simulink model "LCTC_vTD8_Test_TC0_ref6_2007a"  (Simulink 7.0)
settings: Solver=ode4  StartTime=0.0  StopTime=110  FixedStep=0.01  RelTol=1e-3
InitFcn:
  | PedalInterp_para
values from neighbouring files (symbols this model uses):
  ped_min = 5    [PedalInterp_para.m]
  T_max_Brake = 4000    [PedalInterp_para.m]
  TI = 0    [PAS_callback.m]
undefined symbols (not defined in the file or in its folder): fzgbib, m_ab_100pro, m_ab_70pro, PedalInterpretation, v_bereich
libraries: simulink x320
(part 1 of 23)
settings Model: Creator=Justyna  LastModifiedBy=Administrator  ExtModeAutoUpdateStatusClock=off
settings DataIOCC: SaveFormat=StructureWithTime  OutputSaveName=ZZZ
settings DebuggingCC: SaveWithParameterizedLinksMsg=none  SignalResolutionControl=TryResolveAllWithWarning  MultiTaskDSMMsg=warning  MultiTaskCondExecSysMsg=none  StrictBusMsg=None
settings HardwareCC: TargetHWDeviceType=32-bit Generic
settings RTWCC: IncludeERTFirstTime=on
settings GRTTargetCC: TargetFcnLib=ansi_tfl_tmw.mat

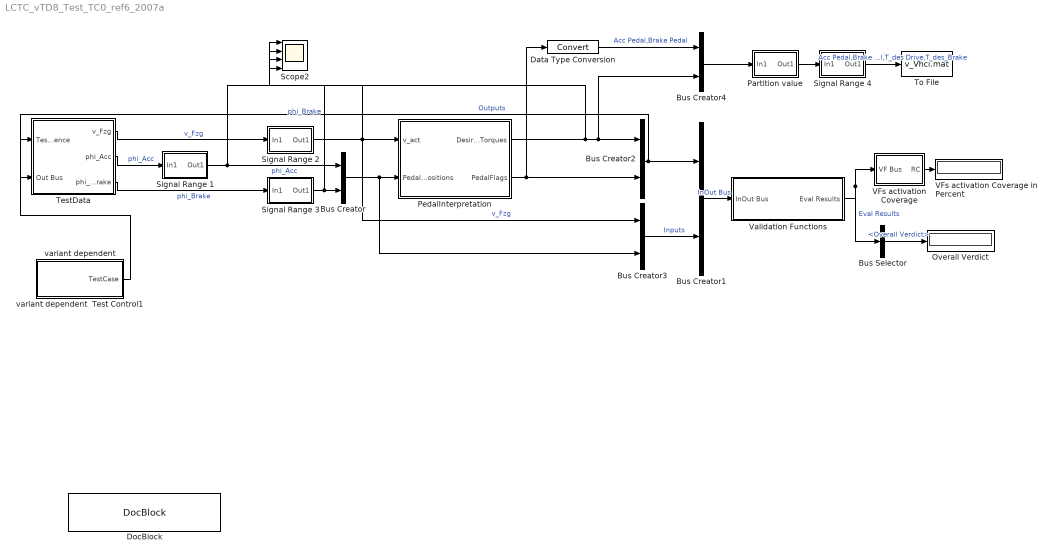
== system LCTC_vTD8_Test_TC0_ref6_2007a ==
  Bus Creator{,1..4} (5 alike) : BusCreator  Inputs=2
  Bus Selector : BusSelector  OutputSignals=Overall Verdict
  Data Type Conversion : DataTypeConversion  OutDataType=sfix(16)  OutScaling=2^0
  DocBlock : simulink/Model-Wide Utilities/DocBlock  SystemSampleTime=-1  DocumentType=Text
      content=|
      | jza - 21.08.07
      | The test model is created manually.
      |
      | Transformation rules for test data variants generation that should be implemented to obtain such a test model automatically are:
      | - for each set of generated variants a Stateflow should be added from the MIL Library: Test Data: Feature generation: Generate feature variants: TestDataVariantsSequence
      | - the number of states (with changed parameters)within TestDataVariantsSequence depends on the number of variants, so the states should be added if missing
      | - after(..) statement within TestDataVariantsSequence should be there as well, however we assume that the time value will be done manually (the same like in the case of independent test control)
      | - please note, that Generate limited increase and Generate limited decrease have been changed, however the same names and the same parameters are used. Probably, there will be no/less adjustment in the current version of transformation.
      | - SR block must contain such kind of brackets [x,y] instad of (x,y)
      |
      | jza - 14.09.07
      | corrections:
      | - switch in variants has a wrong condition - it should be u~=0,
      | - the number in a constant in variants does not work well - it worked for 2, for 3, but not for 4.
      | - time should be a parameter for: td variants, precondition duration, ingredient of test case duration in test control, ingredient of execution time
      | - constant in td have still boolean data type, although it should be "inherited from constant"
  "Overall Verdict   " : Display
  Partition value : Subsystem  mask{sr=[[],[],[0],[0]]}
      mask prompts: sr "signal range"
      mask help: Set the signal range for the input signals. The formal of range is (lower, upper). Lower stands for setting the minimum value of the input signal. Upper stands for setting the maximum value of the input signal. For example (-10,10)
      mask Display: fprintf('SR')
  PedalInterpretation : Subsystem  AncestorBlock=fzgbib/PedalInterpretation
      mask Display: fprintf('SUT')
  Scope2 : Scope  NumInputPorts=4
      settings: TimeRange=72  YMin=0~0~0~0.646597  YMax=70~0.275~27.5~0.908377  SaveName=ScopeData12  MaxDataPoints=11115000
  Signal Range 1 : Subsystem  mask{sr='[0,100]{}'}
      mask prompts: sr "signal range"
      mask help: Set the signal range for the input signals. The formal of range is (lower, upper). Lower stands for setting the minimum value of the input signal. Upper stands for setting the maximum value of the input signal. For example (-10,10)
      mask Display: fprintf('SR')
  Signal Range 2 : Subsystem  mask{sr='[-10,70]{0}'}
      mask prompts: sr "signal range"
      mask help: Set the signal range for the input signals. The formal of range is (lower, upper). Lower stands for setting the minimum value of the input signal. Upper stands for setting the maximum value of the input signal. For example (-10,10)
      mask Display: fprintf('SR')
  Signal Range 3 : Subsystem  mask{sr='[0,100]{}'}
      mask prompts: sr "signal range"
      mask help: Set the signal range for the input signals. The formal of range is (lower, upper). Lower stands for setting the minimum value of the input signal. Upper stands for setting the maximum value of the input signal. For example (-10,10)
      mask Display: fprintf('SR')
  Signal Range 4 : Subsystem  mask{sr=[[0,1],[0,1],[-8000,2300],[0,4000]]}
      mask prompts: sr "signal range"
      mask help: Set the signal range for the input signals. The formal of range is (lower, upper). Lower stands for setting the minimum value of the input signal. Upper stands for setting the maximum value of the input signal. For example (-10,10)
      mask Display: fprintf('SR')
  TestData : Subsystem
  To File : ToFile  Filename=v_Vhcl.mat  MatrixName=v_Vhcl
  VFs activation Coverage : Subsystem  mask{req=11, So=on}
      mask prompts: req "Number of Evaluated Scenarios within Requirements"; So "Adjust to the present Eva Results"
      mask StyleString: popup(1|2|3|4|5|6|7|8|9|10|11|12|13|14|15|16|17|18|19|20),checkbox
      mask CallbackString: |Requirements_Coverage_callback(gcb,-1)
  VFs activation Coverage in Percent : Display
  Validation Functions : Subsystem
  variant dependent : Subsystem  Orientation=left
  variant dependent  Test Control1 : Subsystem
  wires:
  PedalInterpretation/1(DesiredTorques) -> Scope2/3, Bus Creator2/1, Bus Creator4/2
  Bus Creator/1 -> PedalInterpretation/2(PedalPositions), Bus Creator3/2
  PedalInterpretation/2(PedalFlags) -> Bus Creator2/2, Data Type Conversion/1
  Validation Functions/1(Eval Results) -> VFs activation Coverage/1(VF Bus), Bus Selector/1  "Eval Results"
  Bus Creator1/1 -> Validation Functions/1(InOut Bus)  "InOut Bus"
  Bus Creator2/1 -> Bus Creator1/1, TestData/2(Out Bus)  "Outputs"
  Bus Creator3/1 -> Bus Creator1/2  "Inputs"
  VFs activation Coverage/1(RC) -> VFs activation Coverage in Percent/1
  Bus Selector/1 -> "Overall Verdict   "/1  "<Overall Verdict>"
  Signal Range 1/1(Out1) -> Bus Creator/1, Scope2/2  "phi_Acc"
  Signal Range 2/1(Out1) -> PedalInterpretation/1("v_act "), Bus Creator3/1, Scope2/1  "v_Fzg"
  Signal Range 3/1(Out1) -> Bus Creator/2, Scope2/4  "phi_Brake"
  Bus Creator4/1 -> Partition value/1(In1)
  Data Type Conversion/1 -> Bus Creator4/1  "Acc Pedal,Brake Pedal"
  Signal Range 4/1(Out1) -> To File/1  "Acc Pedal,Brake Pedal,T_des Drive,T_des_Brake"
  Partition value/1(Out1) -> Signal Range 4/1(In1)
  TestData/1(v_Fzg) -> Signal Range 2/1(In1)  "v_Fzg"
  TestData/2(phi_Acc) -> Signal Range 1/1(In1)  "phi_Acc"
  TestData/3(phi_Brake) -> Signal Range 3/1(In1)  "phi_Brake"
  variant dependent  Test Control1/1(TestCase) -> TestData/1(Test Ctrl Influence)

== system LCTC_vTD8_Test_TC0_ref6_2007a/Partition value ==
  In1 : Inport  OutDataType=sfix(16)  OutScaling=2^0
  Out1 : Outport  OutDataType=sfix(16)  OutScaling=2^0
  wires:
  In1/1 -> Out1/1

== system LCTC_vTD8_Test_TC0_ref6_2007a/PedalInterpretation ==
  note: 0 ... released
      | 1 ... depressed
  note: T_des_Drive [Nm] (Wunschabtriebsmoment)
      | T_Des_Brake [Nm] (Wunschbremsmoment)
  note: v_act [m/s]
      | (aktuelle Fzg.Längsgeschwindigkeit)
  note: PedalPositions [%]
      | (normierte Pedalwege)
  "v_act " : Inport  OutDataType=sfix(16)  OutScaling=2^0
  PedalPositions : Inport  Port=2  OutDataType=sfix(16)  OutScaling=2^0
  Bus Selector : BusSelector  OutputSignals=phi_Acc,phi_Brake
  Bus Selector1 : BusSelector  OutputSignals=phi_Acc,phi_Brake
  Data Type Conversion : DataTypeConversion  OutDataTypeMode=boolean  OutDataType=sfix(16)  OutScaling=2^0  SaturateOnIntegerOverflow=on  RndMeth=Zero
  Data Type Conversion1 : DataTypeConversion  OutDataTypeMode=boolean  OutDataType=sfix(16)  OutScaling=2^0  SaturateOnIntegerOverflow=on  RndMeth=Zero
  Gain : Gain  Gain=1/70  ParameterDataType=sfix(16)  ParameterScaling=2^0  OutDataType=sfix(16)  OutScaling=2^0  SaturateOnIntegerOverflow=on
  Gain1 : Gain  Gain=1/30  ParameterDataType=sfix(16)  ParameterScaling=2^0  OutDataType=sfix(16)  OutScaling=2^0  SaturateOnIntegerOverflow=on
  Gain2 : Gain  Gain=T_max_Brake  ParameterDataType=sfix(16)  ParameterScaling=2^0  OutDataType=sfix(16)  OutScaling=2^0  SaturateOnIntegerOverflow=on
  Gain3 : Gain  Gain=1/100  ParameterDataType=sfix(16)  ParameterScaling=2^0  OutDataType=sfix(16)  OutScaling=2^0  SaturateOnIntegerOverflow=on
  Mux : Mux  Inputs=2
  Mux1 : Mux  Inputs=3
  Mux3 : Mux  Inputs=2
  Product1 : Product  OutDataType=sfix(16)  OutScaling=2^0  SaturateOnIntegerOverflow=on  InputSameDT=on
  Product2 : Product  OutDataType=sfix(16)  OutScaling=2^0  SaturateOnIntegerOverflow=on  InputSameDT=on
  Relational Operator : RelationalOperator  InputSameDT=on
  Relational Operator1 : RelationalOperator  InputSameDT=on
  Sum : Sum  Inputs=+-  OutDataType=sfix(16)  OutScaling=2^0  SaturateOnIntegerOverflow=on  InputSameDT=on
  Sum1 : Sum  Inputs=+-  OutDataType=sfix(16)  OutScaling=2^0  SaturateOnIntegerOverflow=on  InputSameDT=on
  Sum2 : Sum  OutDataType=sfix(16)  OutScaling=2^0  SaturateOnIntegerOverflow=on  InputSameDT=on
  T_100_Drive(v) : Lookup  InputValues=v_bereich  Table=m_ab_100pro  OutDataType=sfix(16)  OutScaling=2^0  SaturateOnIntegerOverflow=on
  T_70_Drive(v) : Lookup  InputValues=v_bereich  Table=m_ab_70pro  OutDataType=sfix(16)  OutScaling=2^0  SaturateOnIntegerOverflow=on
  Threshold [%] : Constant  Value=ped_min  OutDataType=sfix(16)  OutScaling=2^0
  const : Constant  Value=70  OutDataType=sfix(16)  OutScaling=2^0
  selection : Fcn  Expr=(u(3)>=70)*u(1) +(u(3)<70)*u(2)
  DesiredTorques : Outport  OutDataType=sfix(16)  OutScaling=2^0  InitialOutput=0
  PedalFlags : Outport  Port=2  OutDataType=sfix(16)  OutScaling=2^0  InitialOutput=0
  wires:
  Mux3/1 -> DesiredTorques/1
  Product1/1 -> Gain/1
  T_100_Drive(v)/1 -> Sum/1
  T_70_Drive(v)/1 -> Sum/2, Product1/1, Sum2/2
  Product2/1 -> Sum2/1
  "v_act "/1 -> T_70_Drive(v)/1, T_100_Drive(v)/1  "v_act"
  Gain2/1 -> Gain3/1  "T_des_Brake"
  Bus Selector/2 -> Gain2/1  "<phi_Brake>"
  PedalPositions/1 -> Bus Selector/1, Bus Selector1/1
  Bus Selector/1 -> Product1/2, Sum1/1, Mux1/3  "<phi_Acc>"
  Mux1/1 -> selection/1
  selection/1 -> Mux3/1  "T_des_Drive"
  const/1 -> Sum1/2
  Sum1/1 -> Gain1/1
  Sum/1 -> Product2/2
  Gain1/1 -> Product2/1
  Gain/1 -> Mux1/2
  Sum2/1 -> Mux1/1
  Threshold [%]/1 -> Relational Operator1/2, Relational Operator/2
  Bus Selector1/1 -> Relational Operator/1  "<phi_Acc>"
  Bus Selector1/2 -> Relational Operator1/1  "<phi_Brake>"
  Relational Operator/1 -> Data Type Conversion/1  "AccPedal"
  Relational Operator1/1 -> Data Type Conversion1/1  "BrakePedal"
  Mux/1 -> PedalFlags/1
  Data Type Conversion/1 -> Mux/1  "AccPedal"
  Data Type Conversion1/1 -> Mux/2  "BrakePedal"
  Gain3/1 -> Mux3/2  "T_des_Brake"

== system LCTC_vTD8_Test_TC0_ref6_2007a/Signal Range 1 ==
  In1 : Inport  OutDataType=sfix(16)  OutScaling=2^0
  Out1 : Outport  OutDataType=sfix(16)  OutScaling=2^0
  wires:
  In1/1 -> Out1/1

== system LCTC_vTD8_Test_TC0_ref6_2007a/Signal Range 2 ==
  In1 : Inport  OutDataType=sfix(16)  OutScaling=2^0
  Out1 : Outport  OutDataType=sfix(16)  OutScaling=2^0
  wires:
  In1/1 -> Out1/1

== system LCTC_vTD8_Test_TC0_ref6_2007a/Signal Range 3 ==
  In1 : Inport  OutDataType=sfix(16)  OutScaling=2^0
  Out1 : Outport  OutDataType=sfix(16)  OutScaling=2^0
  wires:
  In1/1 -> Out1/1

== system LCTC_vTD8_Test_TC0_ref6_2007a/Signal Range 4 ==
  In1 : Inport  OutDataType=sfix(16)  OutScaling=2^0
  Out1 : Outport  OutDataType=sfix(16)  OutScaling=2^0
  wires:
  In1/1 -> Out1/1

== system LCTC_vTD8_Test_TC0_ref6_2007a/TestData ==
  Test Ctrl Influence : Inport  OutDataType=sfix(16)  OutScaling=2^0
  Out Bus : Inport  Port=2  OutDataType=sfix(16)  OutScaling=2^0
  Bus Creator 1 : BusCreator  Inputs=12
  Bus Selector phi_Acc : BusSelector  OutputSignals=phi_Acc (signal 2),phi_Acc (signal 5),phi_Acc (signal 8),phi_Acc (signal 11)
  Bus Selector phi_Brake : BusSelector  OutputSignals=phi_Brake (signal 3),phi_Brake (signal 6),phi_Brake (signal 9),phi_Brake (signal 12)
  Bus Selector v_Fzg : BusSelector  OutputSignals=v_Fzg (signal 1),v_Fzg (signal 4),v_Fzg (signal 7),v_Fzg (signal 10)
  PrecAct phi_Acc : MultiPortSwitch  Inputs=5  zeroidx=on
  PrecAct phi_Brake : MultiPortSwitch  Inputs=5  zeroidx=on
  PrecAct v_Fzg : MultiPortSwitch  Inputs=5  zeroidx=on
  SR-PI-01.1 Brake Pedal recognition : Subsystem
  SR-PI-01.3 Acceleration Pedal recognition : Subsystem
  SR-PI-02.1 Brake pedal interpretation : Subsystem
  SR-PI-02.2 Acceleration pedal interpretation : Subsystem
  zero : Constant  Value=0  OutDataType=sfix(16)  OutScaling=2^0
  v_Fzg : Outport  OutDataType=sfix(16)  OutScaling=2^0
  phi_Acc : Outport  Port=2  OutDataType=sfix(16)  OutScaling=2^0
  phi_Brake : Outport  Port=3  OutDataType=sfix(16)  OutScaling=2^0
  wires:
  PrecAct v_Fzg/1 -> v_Fzg/1
  Test Ctrl Influence/1 -> PrecAct v_Fzg/1, PrecAct phi_Acc/1, PrecAct phi_Brake/1
  PrecAct phi_Acc/1 -> phi_Acc/1
  PrecAct phi_Brake/1 -> phi_Brake/1
  zero/1 -> PrecAct v_Fzg/2, PrecAct phi_Acc/2, PrecAct phi_Brake/2
  SR-PI-01.1 Brake Pedal recognition/1(v_Fzg) -> Bus Creator 1/1  "v_Fzg"
  SR-PI-01.1 Brake Pedal recognition/2(phi_Acc) -> Bus Creator 1/2  "phi_Acc"
  SR-PI-01.1 Brake Pedal recognition/3(phi_Brake) -> Bus Creator 1/3  "phi_Brake"
  SR-PI-01.3 Acceleration Pedal recognition/1(v_Fzg) -> Bus Creator 1/4  "v_Fzg"
  SR-PI-01.3 Acceleration Pedal recognition/2(phi_Acc) -> Bus Creator 1/5  "phi_Acc"
  SR-PI-01.3 Acceleration Pedal recognition/3(phi_Brake) -> Bus Creator 1/6  "phi_Brake"
  SR-PI-02.1 Brake pedal interpretation/1(v_Fzg) -> Bus Creator 1/7  "v_Fzg"
  SR-PI-02.1 Brake pedal interpretation/2(phi_Acc) -> Bus Creator 1/8  "phi_Acc"
  SR-PI-02.1 Brake pedal interpretation/3(phi_Brake) -> Bus Creator 1/9  "phi_Brake"
  SR-PI-02.2 Acceleration pedal interpretation/1(v_Fzg) -> Bus Creator 1/10  "v_Fzg"
  SR-PI-02.2 Acceleration pedal interpretation/2(phi_Acc) -> Bus Creator 1/11  "phi_Acc"
  SR-PI-02.2 Acceleration pedal interpretation/3(phi_Brake) -> Bus Creator 1/12  "phi_Brake"
  Bus Creator 1/1 -> Bus Selector v_Fzg/1, Bus Selector phi_Acc/1, Bus Selector phi_Brake/1
  Bus Selector v_Fzg/1 -> PrecAct v_Fzg/3  "<v_Fzg (signal 1)>"
  Bus Selector v_Fzg/2 -> PrecAct v_Fzg/4  "<v_Fzg (signal 4)>"
  Bus Selector v_Fzg/3 -> PrecAct v_Fzg/5  "<v_Fzg (signal 7)>"
  Bus Selector v_Fzg/4 -> PrecAct v_Fzg/6  "<v_Fzg (signal 10)>"
  Bus Selector phi_Acc/1 -> PrecAct phi_Acc/3  "<phi_Acc (signal 2)>"
  Bus Selector phi_Acc/2 -> PrecAct phi_Acc/4  "<phi_Acc (signal 5)>"
  Bus Selector phi_Acc/3 -> PrecAct phi_Acc/5  "<phi_Acc (signal 8)>"
  Bus Selector phi_Acc/4 -> PrecAct phi_Acc/6  "<phi_Acc (signal 11)>"
  Bus Selector phi_Brake/1 -> PrecAct phi_Brake/3  "<phi_Brake (signal 3)>"
  Bus Selector phi_Brake/2 -> PrecAct phi_Brake/4  "<phi_Brake (signal 6)>"
  Bus Selector phi_Brake/3 -> PrecAct phi_Brake/5  "<phi_Brake (signal 9)>"
  Bus Selector phi_Brake/4 -> PrecAct phi_Brake/6  "<phi_Brake (signal 12)>"
  Out Bus/1 -> SR-PI-02.2 Acceleration pedal interpretation/1(Out Bus)

== system LCTC_vTD8_Test_TC0_ref6_2007a/VFs activation Coverage ==
  VF Bus : Inport  OutDataType=sfix(16)  OutScaling=2^0
  Bus Selector : BusSelector  OutputSignals=Local Verdicts.Local verdict (signal 1),Local Verdicts.Local verdict (signal 2),Local Verdicts.Local verdict (signal 3),Local Verdicts.Local verdict (signal 4),Local Verdicts.Local verdict (signal 5),Local Verdicts.Local verdict (signal 6),Local Verdicts.Local verdict (signal 7),Local Verdicts.Local verdict (signal 8),Local Verdicts.Local verdict (signal 9),Local Verdicts.Local verdict (signal 10),Local Verdicts.Local verdict (signal 11)
  Data Type Conversion : DataTypeConversion  OutDataType=sfix(16)  OutScaling=2^0
  Divide : Product  Inputs=*/  OutDataType=sfix(16)  OutScaling=2^-10
  Max to date : Subsystem  TreatAsAtomicUnit=on
  Max to date1 : Subsystem  TreatAsAtomicUnit=on
  Max to date10 : Subsystem  TreatAsAtomicUnit=on
  Max to date2 : Subsystem  TreatAsAtomicUnit=on
  Max to date3 : Subsystem  TreatAsAtomicUnit=on
  Max to date4 : Subsystem  TreatAsAtomicUnit=on
  Max to date5 : Subsystem  TreatAsAtomicUnit=on
  Max to date6 : Subsystem  TreatAsAtomicUnit=on
  Max to date7 : Subsystem  TreatAsAtomicUnit=on
  Max to date8 : Subsystem  TreatAsAtomicUnit=on
  Max to date9 : Subsystem  TreatAsAtomicUnit=on
  Requirements Coverage : Display
  Sum : Sum  Inputs=|+++++++++++  OutDataType=sfix(16)  OutScaling=2^0
  nb of scenarios : Constant  Value=req  OutDataType=sfix(16)  OutScaling=2^0
  percentage : Gain  Gain=100  ParameterDataType=sfix(16)  ParameterScaling=2^0  OutDataType=sfix(16)  OutScaling=2^0
  verdict is  not none{,1..10} (11 alike) : simulink/Logic and Bit Operations/Compare To Constant  SystemSampleTime=-1  relop=~=  const=2  LogicOutDataTypeMode=uint8  ZeroCross=off
  RC : Outport  OutDataType=sfix(16)  OutScaling=2^0
  wires:
  VF Bus/1 -> Bus Selector/1
  Bus Selector/1 -> verdict is  not none/1  "<Local verdict (signal 1)>"
  Bus Selector/2 -> verdict is  not none1/1  "<Local verdict (signal 2)>"
  Bus Selector/3 -> verdict is  not none2/1  "<Local verdict (signal 3)>"
  Bus Selector/4 -> verdict is  not none3/1  "<Local verdict (signal 4)>"
  Bus Selector/5 -> verdict is  not none4/1  "<Local verdict (signal 5)>"
  Bus Selector/6 -> verdict is  not none5/1  "<Local verdict (signal 6)>"
  Bus Selector/7 -> verdict is  not none6/1  "<Local verdict (signal 7)>"
  Bus Selector/8 -> verdict is  not none7/1  "<Local verdict (signal 8)>"
  Bus Selector/9 -> verdict is  not none8/1  "<Local verdict (signal 9)>"
  Sum/1 -> Requirements Coverage/1, Data Type Conversion/1
  percentage/1 -> RC/1
  Max to date/1(Max) -> Sum/1
  Max to date1/1(Max) -> Sum/2
  Max to date2/1(Max) -> Sum/3
  Max to date3/1(Max) -> Sum/4
  Max to date4/1(Max) -> Sum/5
  Max to date5/1(Max) -> Sum/6
  Max to date6/1(Max) -> Sum/7
  Max to date7/1(Max) -> Sum/8
  Max to date8/1(Max) -> Sum/9
  Data Type Conversion/1 -> Divide/1
  verdict is  not none/1 -> Max to date/1(Signal)
  verdict is  not none1/1 -> Max to date1/1(Signal)
  verdict is  not none2/1 -> Max to date2/1(Signal)
  verdict is  not none3/1 -> Max to date3/1(Signal)
  verdict is  not none4/1 -> Max to date4/1(Signal)
  verdict is  not none5/1 -> Max to date5/1(Signal)
  verdict is  not none6/1 -> Max to date6/1(Signal)
  verdict is  not none7/1 -> Max to date7/1(Signal)
  verdict is  not none8/1 -> Max to date8/1(Signal)
  Divide/1 -> percentage/1
  nb of scenarios/1 -> Divide/2
  Bus Selector/10 -> verdict is  not none9/1  "<Local verdict (signal 10)>"
  verdict is  not none9/1 -> Max to date9/1(Signal)
  Max to date9/1(Max) -> Sum/10
  Bus Selector/11 -> verdict is  not none10/1  "<Local verdict (signal 11)>"
  verdict is  not none10/1 -> Max to date10/1(Signal)
  Max to date10/1(Max) -> Sum/11

== system LCTC_vTD8_Test_TC0_ref6_2007a/Validation Functions ==
  InOut Bus : Inport  OutDataType=sfix(16)  OutScaling=2^0
  Arbitration : Subsystem
  Bus Creator : BusCreator
  Bus Creator1 : BusCreator  Inputs=2
  Bus Creator4 : BusCreator  Inputs=11
  Bus Selector : BusSelector  OutputSignals=signal1.signal1.Local verdict,signal1.signal2.Local verdict,signal2.signal1.Local verdict,signal2.signal2.Local verdict,signal3.signal1.Local verdict,signal4.signal1.Local verdict,signal4.signal2.Local verdict,signal4.signal3.Local verdict,signal4.signal4.Local verdict,signal4.signal5.Local verdict,signal4.signal6.Local verdict
  Bus Selector1 : BusSelector  OutputSignals=Inputs.v_Fzg,Inputs.signal2.phi_Acc,Inputs.signal2.phi_Brake,Outputs.signal1.T_des_Drive,Outputs.signal1.T_des_Brake,Outputs.signal2.AccPedal,Outputs.signal2.BrakePedal
  Datatype conversion : Subsystem  TreatAsAtomicUnit=on
  SR-PI-01.1 Brake Pedal recognition : Subsystem
  SR-PI-01.3 Acceleration Pedal recognition : Subsystem
  SR-PI-02.1 Brake pedal interpretation : Subsystem
  SR-PI-02.2 Acceleration pedal interpretation : Subsystem
  Scope1 : Scope  NumInputPorts=4
      settings: TimeRange=140  YMin=0~-1~-5~0.646597  YMax=20~11~5~0.908377  SaveName=ScopeData3  MaxDataPoints=11115000
  Scope2 : Scope  NumInputPorts=5
      settings: TimeRange=72  YMin=0~-5~-5~0.646597~-5  YMax=3~5~5~0.908377~5  SaveName=ScopeData9  MaxDataPoints=11115000
  Scope4 : Scope  NumInputPorts=6
      settings: TimeRange=72  YMin=0~-5~-5~0.646597~-5~-5  YMax=3~5~5~0.908377~5~5  SaveName=ScopeData2  MaxDataPoints=11115000
  Eval Results : Outport  OutDataType=sfix(16)  OutScaling=2^0
  wires:
  InOut Bus/1 -> Datatype conversion/1(InOutBus)
  Bus Creator/1 -> Bus Selector/1
  SR-PI-01.3 Acceleration Pedal recognition/1(Test Info) -> Bus Creator/2
  SR-PI-01.1 Brake Pedal recognition/1(Test Info) -> Bus Creator/1
  SR-PI-02.1 Brake pedal interpretation/1(Test Info) -> Bus Creator/3
  SR-PI-02.2 Acceleration pedal interpretation/1(Test Info) -> Bus Creator/4
  Bus Selector/1 -> Arbitration/1(In1), Bus Creator4/1, Scope2/1  "<Local verdict>"
  Bus Selector/2 -> Arbitration/2(In2), Bus Creator4/2, Scope2/2  "<Local verdict>"
  Bus Selector/3 -> Arbitration/3(In3), Bus Creator4/3, Scope2/3  "<Local verdict>"
  Bus Selector/4 -> Arbitration/4(In4), Bus Creator4/4, Scope2/4  "<Local verdict>"
  Bus Selector/5 -> Arbitration/5(In5), Bus Creator4/5, Scope2/5  "<Local verdict>"
  Bus Selector/6 -> Arbitration/6(In6), Bus Creator4/6, Scope4/1  "<Local verdict>"
  Bus Selector/7 -> Arbitration/7(In7), Bus Creator4/7, Scope4/2  "<Local verdict>"
  Bus Selector/8 -> Arbitration/8(In8), Bus Creator4/8, Scope4/3  "<Local verdict>"
  Bus Selector/9 -> Arbitration/9(In9), Bus Creator4/9, Scope4/4  "<Local verdict>"
  Arbitration/1(Out1) -> Bus Creator1/1  "Overall Verdict"
  Datatype conversion/1(InOut Bus) -> SR-PI-02.1 Brake pedal interpretation/1(InOut Bus), SR-PI-02.2 Acceleration pedal interpretation/1(InOut Bus), Bus Selector1/1, SR-PI-01.3 Acceleration Pedal recognition/1(InOut Bus), SR-PI-01.1 Brake Pedal recognition/1(InOut Bus)
  Bus Creator4/1 -> Bus Creator1/2  "Local Verdicts"
  Bus Creator1/1 -> Eval Results/1
  Bus Selector1/1 -> Scope1/1  "<v_Fzg>"
  Bus Selector1/2 -> Scope1/2  "<phi_Acc>"
  Bus Selector1/3 -> Scope1/3  "<phi_Brake>"
  Bus Selector1/4 -> Scope1/4  "<T_des_Drive>"
  Bus Selector/10 -> Bus Creator4/10, Scope4/5, Arbitration/10(In10)  "<Local verdict>"
  Bus Selector/11 -> Bus Creator4/11, Scope4/6, Arbitration/11(In11)  "<Local verdict>"

== system LCTC_vTD8_Test_TC0_ref6_2007a/variant dependent ==
  variant dependent  Test Control_1 : Stateflow chart  Orientation=left
  TestCase : Outport  OutDataType=sfix(16)  OutScaling=2^0
  tag scope: A=global
  wires:
  variant dependent  Test Control_1/1(TestCase) -> TestCase/1  "TestCase"
  variant dependent  Test Control_1/2(variant) -> [A]

== system LCTC_vTD8_Test_TC0_ref6_2007a/variant dependent  Test Control1 ==
  variant dependent  Test Control : Stateflow chart  Orientation=left
  TestCase : Outport  OutDataType=sfix(16)  OutScaling=2^0
  tag scope: variant=global
  wires:
  variant dependent  Test Control/1(TestCase) -> TestCase/1
  variant dependent  Test Control/2(variant) -> [variant]

== system LCTC_vTD8_Test_TC0_ref6_2007a/TestData/SR-PI-01.1 Brake Pedal recognition ==
  Bus Creator 1 : BusCreator  Inputs=2
  Bus Selector phi_Brake : BusSelector  OutputSignals=phi_Brake (signal 1),phi_Brake (signal 2)
  Initialisation & Stabilisation : Subsystem
  PrecAct phi_Brake : MultiPortSwitch  Inputs=3
  Sequencing of test data in time due to Preconditions : Stateflow chart
  phi_Acc random : Constant  Value=0  OutDataType=sfix(16)  OutScaling=2^0
  phi_Brake < ped_min : Subsystem
  phi_Brake >= ped_min : Subsystem
  v_Fzg random : Constant  Value=0  OutDataType=sfix(16)  OutScaling=2^0
  v_Fzg : Outport  OutDataType=sfix(16)  OutScaling=2^0
  phi_Acc : Outport  Port=2  OutDataType=sfix(16)  OutScaling=2^0
  phi_Brake : Outport  Port=3  OutDataType=sfix(16)  OutScaling=2^0
  wires:
  Sequencing of test data in time due to Preconditions/1(TDPre) -> PrecAct phi_Brake/1
  PrecAct phi_Brake/1 -> phi_Brake/1
  phi_Brake < ped_min/1(phi_Brake) -> Bus Creator 1/1  "phi_Brake"
  phi_Brake >= ped_min/1(phi_Brake) -> Bus Creator 1/2  "phi_Brake"
  Bus Creator 1/1 -> Bus Selector phi_Brake/1
  Bus Selector phi_Brake/1 -> PrecAct phi_Brake/2  "<phi_Brake (signal 1)>"
  Bus Selector phi_Brake/2 -> PrecAct phi_Brake/3  "<phi_Brake (signal 2)>"
  v_Fzg random/1 -> v_Fzg/1  "v_Fzg"
  phi_Acc random/1 -> phi_Acc/1  "phi_Acc"
  Initialisation & Stabilisation/3(phi_Brake neutral) -> PrecAct phi_Brake/4  "phi_Brake neutral"

== system LCTC_vTD8_Test_TC0_ref6_2007a/TestData/SR-PI-01.3 Acceleration Pedal recognition ==
  Bus Creator 1 : BusCreator  Inputs=2
  Bus Selector phi_Acc : BusSelector  OutputSignals=phi_Acc (signal 1),phi_Acc (signal 2)
  Initialisation & Stabilisation : Subsystem
  PrecAct phi_Acc : MultiPortSwitch  Inputs=3
  Sequencing of test data in time due to Preconditions : Stateflow chart
  phi_Acc < ped_min : Subsystem
  phi_Acc >= ped_min : Subsystem
  phi_Brake random : Constant  Value=0  OutDataType=sfix(16)  OutScaling=2^0
  v_Fzg random : Constant  Value=0  OutDataType=sfix(16)  OutScaling=2^0
  v_Fzg : Outport  OutDataType=sfix(16)  OutScaling=2^0
  phi_Acc : Outport  Port=2  OutDataType=sfix(16)  OutScaling=2^0
  phi_Brake : Outport  Port=3  OutDataType=sfix(16)  OutScaling=2^0
  wires:
  PrecAct phi_Acc/1 -> phi_Acc/1
  Sequencing of test data in time due to Preconditions/1(TDPre) -> PrecAct phi_Acc/1
  phi_Acc < ped_min/1(phi_Acc) -> Bus Creator 1/1  "phi_Acc"
  phi_Acc >= ped_min/1(phi_Acc) -> Bus Creator 1/2  "phi_Acc"
  Bus Creator 1/1 -> Bus Selector phi_Acc/1
  Bus Selector phi_Acc/1 -> PrecAct phi_Acc/2  "<phi_Acc (signal 1)>"
  Bus Selector phi_Acc/2 -> PrecAct phi_Acc/3  "<phi_Acc (signal 2)>"
  v_Fzg random/1 -> v_Fzg/1  "v_Fzg"
  Initialisation & Stabilisation/2(phi_Acc neutral) -> PrecAct phi_Acc/4  "phi_Acc neutral"
  phi_Brake random/1 -> phi_Brake/1  "phi_Brake"

== system LCTC_vTD8_Test_TC0_ref6_2007a/TestData/SR-PI-02.1 Brake pedal interpretation ==
  Bus Creator 1 : BusCreator  Inputs=3
  Bus Selector phi_Acc : BusSelector  OutputSignals=phi_Acc
  Bus Selector phi_Brake : BusSelector  OutputSignals=phi_Brake
  Bus Selector v_Fzg : BusSelector  OutputSignals=v_Fzg
  Initialisation & Stabilisation : Subsystem
  PrecAct phi_Acc : MultiPortSwitch  Inputs=2
  PrecAct phi_Brake : MultiPortSwitch  Inputs=2
  PrecAct v_Fzg : MultiPortSwitch  Inputs=2
  Scope2 : Scope  NumInputPorts=4
      settings: TimeRange=72  YMin=-1~-1~-1~-1  YMax=1~1~1~1  MaxDataPoints=11115000
  Sequencing of test data in time due to Preconditions : Stateflow chart
  true : Subsystem
  v_Fzg : Outport  OutDataType=sfix(16)  OutScaling=2^0
  phi_Acc : Outport  Port=2  OutDataType=sfix(16)  OutScaling=2^0
  phi_Brake : Outport  Port=3  OutDataType=sfix(16)  OutScaling=2^0
  wires:
  PrecAct v_Fzg/1 -> v_Fzg/1, Scope2/1
  Sequencing of test data in time due to Preconditions/1(TDPre) -> PrecAct v_Fzg/1, PrecAct phi_Acc/1, PrecAct phi_Brake/1
  PrecAct phi_Acc/1 -> phi_Acc/1, Scope2/2
  PrecAct phi_Brake/1 -> phi_Brake/1, Scope2/3
  true/1(v_Fzg) -> Bus Creator 1/1  "v_Fzg"
  true/2(phi_Acc) -> Bus Creator 1/2  "phi_Acc"
  true/3(phi_Brake) -> Bus Creator 1/3  "phi_Brake"
  Bus Creator 1/1 -> Bus Selector v_Fzg/1, Bus Selector phi_Acc/1, Bus Selector phi_Brake/1
  Bus Selector v_Fzg/1 -> PrecAct v_Fzg/2  "<v_Fzg>"
  Bus Selector phi_Acc/1 -> PrecAct phi_Acc/2  "<phi_Acc>"
  Bus Selector phi_Brake/1 -> PrecAct phi_Brake/2  "<phi_Brake>"
  Initialisation & Stabilisation/1(v_Fzg neutral) -> PrecAct v_Fzg/3  "v_Fzg neutral"
  Initialisation & Stabilisation/2(phi_Acc neutral) -> PrecAct phi_Acc/3  "phi_Acc neutral"
  Initialisation & Stabilisation/3(phi_Brake neutral) -> PrecAct phi_Brake/3  "phi_Brake neutral"

== system LCTC_vTD8_Test_TC0_ref6_2007a/TestData/SR-PI-02.2 Acceleration pedal interpretation ==
  Out Bus : Inport  OutDataType=sfix(16)  OutScaling=2^0
  Bus Creator 1 : BusCreator  Inputs=17
  Bus Selector Seq : BusSelector  OutputSignals=Activate (signal 3),Activate (signal 6),Activate (signal 9),Activate (signal 12),Activate (signal 15)
  Bus Selector phi_Acc : BusSelector  OutputSignals=phi_Acc (signal 2),phi_Acc (signal 5),phi_Acc (signal 8),phi_Acc (signal 11),phi_Acc (signal 14),phi_Acc (signal 16)
  Bus Selector v_Fzg : BusSelector  OutputSignals=v_Fzg (signal 1),v_Fzg (signal 4),v_Fzg (signal 7),v_Fzg (signal 10),v_Fzg (signal 13),v_Fzg (signal 17)
  Initialisation & Stabilisation : Subsystem
  PrecAct phi_Acc : MultiPortSwitch  Inputs=7
  PrecAct v_Fzg : MultiPortSwitch  Inputs=7
  Sequencing of test data in time due to Preconditions : Stateflow chart
  phi_Brake random : Constant  Value=0  OutDataType=sfix(16)  OutScaling=2^0
  v = const & phi_Acc = const : Subsystem
  v = const & phi_Acc decreases & T_des_Drive < 0 : Subsystem
  v = const & phi_Acc decreases & T_des_Drive >= 0 : Subsystem
  v = const & phi_Acc increases & T_des_Drive < 0 : Subsystem
  v = const & phi_Acc increases & T_des_Drive >= 0 : Subsystem
  v increases & phi_Acc = const & T_des_Drive >= 0 : Subsystem
  v_Fzg : Outport  OutDataType=sfix(16)  OutScaling=2^0
  phi_Acc : Outport  Port=2  OutDataType=sfix(16)  OutScaling=2^0
  phi_Brake : Outport  Port=3  OutDataType=sfix(16)  OutScaling=2^0
  wires:
  PrecAct phi_Acc/1 -> phi_Acc/1
  Sequencing of test data in time due to Preconditions/1(TDPre) -> PrecAct phi_Acc/1, PrecAct v_Fzg/1
  PrecAct v_Fzg/1 -> v_Fzg/1
  v = const & phi_Acc = const/1(v_Fzg) -> Bus Creator 1/1  "v_Fzg"
  v = const & phi_Acc = const/2(phi_Acc) -> Bus Creator 1/2  "phi_Acc"
  v = const & phi_Acc decreases & T_des_Drive < 0/1(Activate) -> Bus Creator 1/3  "Activate"
  v = const & phi_Acc decreases & T_des_Drive < 0/2(v_Fzg) -> Bus Creator 1/4  "v_Fzg"
  v = const & phi_Acc decreases & T_des_Drive < 0/3(phi_Acc) -> Bus Creator 1/5  "phi_Acc"
  Out Bus/1 -> v = const & phi_Acc decreases & T_des_Drive < 0/1(Out Bus), v = const & phi_Acc decreases & T_des_Drive >= 0/1(Out Bus), v = const & phi_Acc increases & T_des_Drive < 0/1(Out Bus), v = const & phi_Acc increases & T_des_Drive >= 0/1(Out Bus), v increases & phi_Acc = const & T_des_Drive >= 0/1(Out Bus)
  v = const & phi_Acc decreases & T_des_Drive >= 0/1(Activate) -> Bus Creator 1/6  "Activate"
  v = const & phi_Acc decreases & T_des_Drive >= 0/2(v_Fzg) -> Bus Creator 1/7  "v_Fzg"
  v = const & phi_Acc decreases & T_des_Drive >= 0/3(phi_Acc) -> Bus Creator 1/8  "phi_Acc"
  v = const & phi_Acc increases & T_des_Drive < 0/1(Activate) -> Bus Creator 1/9  "Activate"
  v = const & phi_Acc increases & T_des_Drive < 0/2(v_Fzg) -> Bus Creator 1/10  "v_Fzg"
  v = const & phi_Acc increases & T_des_Drive < 0/3(phi_Acc) -> Bus Creator 1/11  "phi_Acc"
  v = const & phi_Acc increases & T_des_Drive >= 0/1(Activate) -> Bus Creator 1/12  "Activate"
  v = const & phi_Acc increases & T_des_Drive >= 0/2(v_Fzg) -> Bus Creator 1/13  "v_Fzg"
  v = const & phi_Acc increases & T_des_Drive >= 0/3(phi_Acc) -> Bus Creator 1/14  "phi_Acc"
  v increases & phi_Acc = const & T_des_Drive >= 0/1(Activate) -> Bus Creator 1/15  "Activate"
  v increases & phi_Acc = const & T_des_Drive >= 0/2(phi_Acc) -> Bus Creator 1/16  "phi_Acc"
  v increases & phi_Acc = const & T_des_Drive >= 0/3(v_Fzg) -> Bus Creator 1/17  "v_Fzg"
  Bus Creator 1/1 -> Bus Selector v_Fzg/1, Bus Selector phi_Acc/1, Bus Selector Seq/1
  Bus Selector v_Fzg/1 -> PrecAct v_Fzg/2  "<v_Fzg (signal 1)>"
  Bus Selector v_Fzg/2 -> PrecAct v_Fzg/3  "<v_Fzg (signal 4)>"
  Bus Selector v_Fzg/3 -> PrecAct v_Fzg/4  "<v_Fzg (signal 7)>"
  Bus Selector v_Fzg/4 -> PrecAct v_Fzg/5  "<v_Fzg (signal 10)>"
  Bus Selector v_Fzg/5 -> PrecAct v_Fzg/6  "<v_Fzg (signal 13)>"
  Bus Selector v_Fzg/6 -> PrecAct v_Fzg/7  "<v_Fzg (signal 17)>"
  Bus Selector phi_Acc/1 -> PrecAct phi_Acc/2  "<phi_Acc (signal 2)>"
  Bus Selector phi_Acc/2 -> PrecAct phi_Acc/3  "<phi_Acc (signal 5)>"
  Bus Selector phi_Acc/3 -> PrecAct phi_Acc/4  "<phi_Acc (signal 8)>"
  Bus Selector phi_Acc/4 -> PrecAct phi_Acc/5  "<phi_Acc (signal 11)>"
  Bus Selector phi_Acc/5 -> PrecAct phi_Acc/6  "<phi_Acc (signal 14)>"
  Bus Selector phi_Acc/6 -> PrecAct phi_Acc/7  "<phi_Acc (signal 16)>"
  Initialisation & Stabilisation/1(v_Fzg neutral) -> PrecAct v_Fzg/8  "v_Fzg neutral"
  Initialisation & Stabilisation/2(phi_Acc neutral) -> PrecAct phi_Acc/8  "phi_Acc neutral"
  phi_Brake random/1 -> phi_Brake/1  "phi_Brake"
  Bus Selector Seq/1 -> Sequencing of test data in time due to Preconditions/2(Activate2)  "<Activate (signal 3)>"
  Bus Selector Seq/2 -> Sequencing of test data in time due to Preconditions/3(Activate3)  "<Activate (signal 6)>"
  Bus Selector Seq/3 -> Sequencing of test data in time due to Preconditions/6(Activate6)  "<Activate (signal 9)>"
  Bus Selector Seq/4 -> Sequencing of test data in time due to Preconditions/5(Activate5)  "<Activate (signal 12)>"
  Bus Selector Seq/5 -> Sequencing of test data in time due to Preconditions/4(Activate4)  "<Activate (signal 15)>"

== system LCTC_vTD8_Test_TC0_ref6_2007a/VFs activation Coverage/Max to date ==
  Signal : Inport  OutDataType=sfix(16)  OutScaling=2^0
  Clock : Clock
      settings: Decimation=10
  Memory : Memory  Orientation=left
  MinMax : MinMax  Function=max  Inputs=2  OutDataType=sfix(16)  OutScaling=2^0
  Switch : Switch  Criteria=u2 > Threshold
  Max : Outport  OutDataType=sfix(16)  OutScaling=2^0
  wires:
  Memory/1 -> Switch/1
  Clock/1 -> Switch/2
  Switch/1 -> MinMax/1
  Signal/1 -> Switch/3, MinMax/2
  MinMax/1 -> Memory/1, Max/1

== system LCTC_vTD8_Test_TC0_ref6_2007a/VFs activation Coverage/Max to date1 ==
  Signal : Inport  OutDataType=sfix(16)  OutScaling=2^0
  Clock : Clock
      settings: Decimation=10
  Memory : Memory  Orientation=left
  MinMax : MinMax  Function=max  Inputs=2  OutDataType=sfix(16)  OutScaling=2^0
  Switch : Switch  Criteria=u2 > Threshold
  Max : Outport  OutDataType=sfix(16)  OutScaling=2^0
  wires:
  Memory/1 -> Switch/1
  Clock/1 -> Switch/2
  Switch/1 -> MinMax/1
  Signal/1 -> Switch/3, MinMax/2
  MinMax/1 -> Memory/1, Max/1

== system LCTC_vTD8_Test_TC0_ref6_2007a/VFs activation Coverage/Max to date10 ==
  Signal : Inport  OutDataType=sfix(16)  OutScaling=2^0
  Clock : Clock
      settings: Decimation=10
  Memory : Memory  Orientation=left
  MinMax : MinMax  Function=max  Inputs=2  OutDataType=sfix(16)  OutScaling=2^0
  Switch : Switch  Criteria=u2 > Threshold
  Max : Outport  OutDataType=sfix(16)  OutScaling=2^0
  wires:
  MinMax/1 -> Max/1, Memory/1
  Signal/1 -> MinMax/2, Switch/3
  Switch/1 -> MinMax/1
  Clock/1 -> Switch/2
  Memory/1 -> Switch/1

== system LCTC_vTD8_Test_TC0_ref6_2007a/VFs activation Coverage/Max to date2 ==
  Signal : Inport  OutDataType=sfix(16)  OutScaling=2^0
  Clock : Clock
      settings: Decimation=10
  Memory : Memory  Orientation=left
  MinMax : MinMax  Function=max  Inputs=2  OutDataType=sfix(16)  OutScaling=2^0
  Switch : Switch  Criteria=u2 > Threshold
  Max : Outport  OutDataType=sfix(16)  OutScaling=2^0
  wires:
  Memory/1 -> Switch/1
  Clock/1 -> Switch/2
  Switch/1 -> MinMax/1
  Signal/1 -> Switch/3, MinMax/2
  MinMax/1 -> Memory/1, Max/1

== system LCTC_vTD8_Test_TC0_ref6_2007a/VFs activation Coverage/Max to date3 ==
  Signal : Inport  OutDataType=sfix(16)  OutScaling=2^0
  Clock : Clock
      settings: Decimation=10
  Memory : Memory  Orientation=left
  MinMax : MinMax  Function=max  Inputs=2  OutDataType=sfix(16)  OutScaling=2^0
  Switch : Switch  Criteria=u2 > Threshold
  Max : Outport  OutDataType=sfix(16)  OutScaling=2^0
  wires:
  Memory/1 -> Switch/1
  Clock/1 -> Switch/2
  Switch/1 -> MinMax/1
  Signal/1 -> Switch/3, MinMax/2
  MinMax/1 -> Memory/1, Max/1

== system LCTC_vTD8_Test_TC0_ref6_2007a/VFs activation Coverage/Max to date4 ==
  Signal : Inport  OutDataType=sfix(16)  OutScaling=2^0
  Clock : Clock
      settings: Decimation=10
  Memory : Memory  Orientation=left
  MinMax : MinMax  Function=max  Inputs=2  OutDataType=sfix(16)  OutScaling=2^0
  Switch : Switch  Criteria=u2 > Threshold
  Max : Outport  OutDataType=sfix(16)  OutScaling=2^0
  wires:
  Memory/1 -> Switch/1
  Clock/1 -> Switch/2
  Switch/1 -> MinMax/1
  Signal/1 -> Switch/3, MinMax/2
  MinMax/1 -> Memory/1, Max/1

== system LCTC_vTD8_Test_TC0_ref6_2007a/VFs activation Coverage/Max to date5 ==
  Signal : Inport  OutDataType=sfix(16)  OutScaling=2^0
  Clock : Clock
      settings: Decimation=10
  Memory : Memory  Orientation=left
  MinMax : MinMax  Function=max  Inputs=2  OutDataType=sfix(16)  OutScaling=2^0
  Switch : Switch  Criteria=u2 > Threshold
  Max : Outport  OutDataType=sfix(16)  OutScaling=2^0
  wires:
  Memory/1 -> Switch/1
  Clock/1 -> Switch/2
  Switch/1 -> MinMax/1
  Signal/1 -> Switch/3, MinMax/2
  MinMax/1 -> Memory/1, Max/1

== system LCTC_vTD8_Test_TC0_ref6_2007a/VFs activation Coverage/Max to date6 ==
  Signal : Inport  OutDataType=sfix(16)  OutScaling=2^0
  Clock : Clock
      settings: Decimation=10
  Memory : Memory  Orientation=left
  MinMax : MinMax  Function=max  Inputs=2  OutDataType=sfix(16)  OutScaling=2^0
  Switch : Switch  Criteria=u2 > Threshold
  Max : Outport  OutDataType=sfix(16)  OutScaling=2^0
  wires:
  Memory/1 -> Switch/1
  Clock/1 -> Switch/2
  Switch/1 -> MinMax/1
  Signal/1 -> Switch/3, MinMax/2
  MinMax/1 -> Memory/1, Max/1

== system LCTC_vTD8_Test_TC0_ref6_2007a/VFs activation Coverage/Max to date7 ==
  Signal : Inport  OutDataType=sfix(16)  OutScaling=2^0
  Clock : Clock
      settings: Decimation=10
  Memory : Memory  Orientation=left
  MinMax : MinMax  Function=max  Inputs=2  OutDataType=sfix(16)  OutScaling=2^0
  Switch : Switch  Criteria=u2 > Threshold
  Max : Outport  OutDataType=sfix(16)  OutScaling=2^0
  wires:
  Memory/1 -> Switch/1
  Clock/1 -> Switch/2
  Switch/1 -> MinMax/1
  Signal/1 -> Switch/3, MinMax/2
  MinMax/1 -> Memory/1, Max/1

== system LCTC_vTD8_Test_TC0_ref6_2007a/VFs activation Coverage/Max to date8 ==
  Signal : Inport  OutDataType=sfix(16)  OutScaling=2^0
  Clock : Clock
      settings: Decimation=10
  Memory : Memory  Orientation=left
  MinMax : MinMax  Function=max  Inputs=2  OutDataType=sfix(16)  OutScaling=2^0
  Switch : Switch  Criteria=u2 > Threshold
  Max : Outport  OutDataType=sfix(16)  OutScaling=2^0
  wires:
  Memory/1 -> Switch/1
  Clock/1 -> Switch/2
  Switch/1 -> MinMax/1
  Signal/1 -> Switch/3, MinMax/2
  MinMax/1 -> Memory/1, Max/1

== system LCTC_vTD8_Test_TC0_ref6_2007a/VFs activation Coverage/Max to date9 ==
  Signal : Inport  OutDataType=sfix(16)  OutScaling=2^0
  Clock : Clock
      settings: Decimation=10
  Memory : Memory  Orientation=left
  MinMax : MinMax  Function=max  Inputs=2  OutDataType=sfix(16)  OutScaling=2^0
  Switch : Switch  Criteria=u2 > Threshold
  Max : Outport  OutDataType=sfix(16)  OutScaling=2^0
  wires:
  MinMax/1 -> Max/1, Memory/1
  Signal/1 -> MinMax/2, Switch/3
  Switch/1 -> MinMax/1
  Clock/1 -> Switch/2
  Memory/1 -> Switch/1

== system LCTC_vTD8_Test_TC0_ref6_2007a/Validation Functions/Arbitration ==
  In1 : Inport  OutDataType=sfix(16)  OutScaling=2^0
  In2 : Inport  Port=2  OutDataType=sfix(16)  OutScaling=2^0
  In3 : Inport  Port=3  OutDataType=sfix(16)  OutScaling=2^0
  In4 : Inport  Port=4  OutDataType=sfix(16)  OutScaling=2^0
  In5 : Inport  Port=5  OutDataType=sfix(16)  OutScaling=2^0
  In6 : Inport  Port=6  OutDataType=sfix(16)  OutScaling=2^0
  In7 : Inport  Port=7  OutDataType=sfix(16)  OutScaling=2^0
  In8 : Inport  Port=8  OutDataType=sfix(16)  OutScaling=2^0
  In9 : Inport  Port=9  OutDataType=sfix(16)  OutScaling=2^0
  In10 : Inport  Port=10  OutDataType=sfix(16)  OutScaling=2^0
  In11 : Inport  Port=11  OutDataType=sfix(16)  OutScaling=2^0
  Collect Verdicts : MinMax  Inputs=12  OutDataType=sfix(16)  OutScaling=2^0
  Memory : Memory  Orientation=left  X0=2
  Out1 : Outport  OutDataType=sfix(16)  OutScaling=2^0
  wires:
  Memory/1 -> Collect Verdicts/12
  In1/1 -> Collect Verdicts/1
  In2/1 -> Collect Verdicts/2
  In3/1 -> Collect Verdicts/3
  In4/1 -> Collect Verdicts/4
  In5/1 -> Collect Verdicts/5
  Collect Verdicts/1 -> Out1/1, Memory/1
  In6/1 -> Collect Verdicts/6
  In7/1 -> Collect Verdicts/7
  In8/1 -> Collect Verdicts/8
  In9/1 -> Collect Verdicts/9
  In10/1 -> Collect Verdicts/10
  In11/1 -> Collect Verdicts/11

== system LCTC_vTD8_Test_TC0_ref6_2007a/Validation Functions/Datatype conversion ==
  InOutBus : Inport  OutDataType=sfix(16)  OutScaling=2^0
  Bus Creator{,1..5} (6 alike) : BusCreator  Inputs=2
  Bus Selector : BusSelector  OutputSignals=Inputs,Outputs
  Bus Selector1 : BusSelector  OutputSignals=v_Fzg,signal2
  Bus Selector2 : BusSelector  OutputSignals=signal1,signal2
  Bus Selector3 : BusSelector  OutputSignals=phi_Acc,phi_Brake
  Bus Selector4 : BusSelector  OutputSignals=T_des_Drive,T_des_Brake
  Bus Selector5 : BusSelector  OutputSignals=AccPedal,BrakePedal
  Data Type Conversion{,1..6} (7 alike) : DataTypeConversion  OutDataType=sfix(16)  OutScaling=2^0
  InOut Bus : Outport  OutDataType=sfix(16)  OutScaling=2^0
  wires:
  InOutBus/1 -> Bus Selector/1
  Bus Selector/1 -> Bus Selector1/1  "<Inputs>"
  Bus Selector/2 -> Bus Selector2/1  "<Outputs>"
  Bus Selector1/2 -> Bus Selector3/1  "<signal2>"
  Bus Selector2/1 -> Bus Selector4/1  "<signal1>"
  Bus Selector2/2 -> Bus Selector5/1  "<signal2>"
  Bus Selector1/1 -> Data Type Conversion/1  "<v_Fzg>"
  Bus Selector3/1 -> Data Type Conversion1/1  "<phi_Acc>"
  Bus Selector3/2 -> Data Type Conversion2/1  "<phi_Brake>"
  Bus Selector4/1 -> Data Type Conversion3/1  "<T_des_Drive>"
  Bus Selector4/2 -> Data Type Conversion4/1  "<T_des_Brake>"
  Bus Selector5/1 -> Data Type Conversion5/1  "<AccPedal>"
  Bus Selector5/2 -> Data Type Conversion6/1  "<BrakePedal>"
  Data Type Conversion3/1 -> Bus Creator/1  "T_des_Drive"
  Data Type Conversion4/1 -> Bus Creator/2  "T_des_Brake"
  Data Type Conversion5/1 -> Bus Creator1/1  "AccPedal"
  Data Type Conversion6/1 -> Bus Creator1/2  "BrakePedal"
  Data Type Conversion1/1 -> Bus Creator2/1  "phi_Acc"
  Data Type Conversion2/1 -> Bus Creator2/2  "phi_Brake"
  Bus Creator2/1 -> Bus Creator3/2  "signal2"
  Data Type Conversion/1 -> Bus Creator3/1  "v_Fzg"
  Bus Creator/1 -> Bus Creator4/1
  Bus Creator1/1 -> Bus Creator4/2
  Bus Creator3/1 -> Bus Creator5/1  "Inputs"
  Bus Creator4/1 -> Bus Creator5/2  "Outputs"
  Bus Creator5/1 -> InOut Bus/1  "InOutBus"

== system LCTC_vTD8_Test_TC0_ref6_2007a/Validation Functions/SR-PI-01.1 Brake Pedal recognition ==
  InOut Bus : Inport  OutDataType=sfix(16)  OutScaling=2^0
  BrakePedal == 0 : Subsystem  TreatAsAtomicUnit=on
  BrakePedal == 1 : Subsystem  TreatAsAtomicUnit=on
  Bus Creator : BusCreator  Inputs=2
  phi_Brake < ped_min : Subsystem
  phi_Brake >= ped_min : Subsystem
  Test Info : Outport  OutDataType=sfix(16)  OutScaling=2^0
  wires:
  phi_Brake >= ped_min/1(Activate) -> BrakePedal == 1/1(Activate)
  InOut Bus/1 -> phi_Brake >= ped_min/1(InOut Bus), phi_Brake < ped_min/1(InOut Bus), BrakePedal == 1/2(InOut Bus), BrakePedal == 0/2(InOut Bus)
  phi_Brake < ped_min/1(Activate) -> BrakePedal == 0/1(Activate)
  Bus Creator/1 -> Test Info/1
  BrakePedal == 1/1(VF info) -> Bus Creator/1
  BrakePedal == 0/1(VF info) -> Bus Creator/2

== system LCTC_vTD8_Test_TC0_ref6_2007a/Validation Functions/SR-PI-01.3 Acceleration Pedal recognition ==
  InOut Bus : Inport  OutDataType=sfix(16)  OutScaling=2^0
  AccPedal == 0 : Subsystem  TreatAsAtomicUnit=on
  AccPedal == 1 : Subsystem  TreatAsAtomicUnit=on
  Bus Creator : BusCreator  Inputs=2
  phi_Acc < ped_min : Subsystem
  phi_Acc >= ped_min : Subsystem
  Test Info : Outport  OutDataType=sfix(16)  OutScaling=2^0
  wires:
  phi_Acc < ped_min/1(Activate) -> AccPedal == 0/1(Activate)
  InOut Bus/1 -> phi_Acc >= ped_min/1(InOut Bus), phi_Acc < ped_min/1(InOut Bus), AccPedal == 0/2(InOut Bus), AccPedal == 1/2(InOut Bus)
  AccPedal == 1/1(VF info) -> Bus Creator/1
  AccPedal == 0/1(VF info) -> Bus Creator/2
  Bus Creator/1 -> Test Info/1
  phi_Acc >= ped_min/1(Activate) -> AccPedal == 1/1(Activate)

== system LCTC_vTD8_Test_TC0_ref6_2007a/Validation Functions/SR-PI-02.1 Brake pedal interpretation ==
  InOut Bus : Inport  OutDataType=sfix(16)  OutScaling=2^0
  Bus Creator : BusCreator  Inputs=1
  phi_Brake/100 = T_des_Brake/T_max_Brake : Subsystem  TreatAsAtomicUnit=on
  true : Subsystem
  Test Info : Outport  OutDataType=sfix(16)  OutScaling=2^0
  wires:
  InOut Bus/1 -> true/1(InOut Bus), phi_Brake/100 = T_des_Brake/T_max_Brake/2(InOut Bus)
  true/1(Activate) -> phi_Brake/100 = T_des_Brake/T_max_Brake/1(Activate)
  Bus Creator/1 -> Test Info/1
  phi_Brake/100 = T_des_Brake/T_max_Brake/1(VF info) -> Bus Creator/1

== system LCTC_vTD8_Test_TC0_ref6_2007a/Validation Functions/SR-PI-02.2 Acceleration pedal interpretation ==
  InOut Bus : Inport  OutDataType=sfix(16)  OutScaling=2^0
  Bus Creator : BusCreator  Inputs=6
  T_des_Drive = const : Subsystem  TreatAsAtomicUnit=on
  T_des_Drive decreases : Subsystem  TreatAsAtomicUnit=on
  "T_des_Drive decreases " : Subsystem  TreatAsAtomicUnit=on
  T_des_Drive does not increase : Subsystem  TreatAsAtomicUnit=on
  T_des_Drive increases : Subsystem  TreatAsAtomicUnit=on
  "T_des_Drive increases " : Subsystem  TreatAsAtomicUnit=on
  v = const & phi_Acc = const : Subsystem
  v = const & phi_Acc decreases & T_des_Drive < 0 : Subsystem
  v = const & phi_Acc decreases & T_des_Drive >= 0 : Subsystem
  v = const & phi_Acc increases & T_des_Drive < 0 : Subsystem
  v = const & phi_Acc increases & T_des_Drive >= 0 : Subsystem
  v increases & phi_Acc = const & T_des_Drive >= 0 : Subsystem
  Test Info : Outport  OutDataType=sfix(16)  OutScaling=2^0
  wires:
  v = const & phi_Acc increases & T_des_Drive >= 0/1(Activate) -> T_des_Drive increases/1(Activate)
  InOut Bus/1 -> v = const & phi_Acc increases & T_des_Drive >= 0/1(InOut Bus), T_des_Drive increases/2(InOut Bus), v = const & phi_Acc decreases & T_des_Drive >= 0/1(InOut Bus), v = const & phi_Acc = const/1(InOut Bus), v increases & phi_Acc = const & T_des_Drive >= 0/1(InOut Bus), T_des_Drive does not increase/2(InOut Bus), v = const & phi_Acc increases & T_des_Drive < 0/1(InOut Bus), "T_des_Drive decreases "/2(InOut Bus), v = const & phi_Acc decreases & T_des_Drive < 0/1(InOut Bus), "T_des_Drive increases "/2(InOut Bus), T_des_Drive = const/2(InOut Bus), T_des_Drive decreases/2(InOut Bus)
  v = const & phi_Acc decreases & T_des_Drive >= 0/1(Activate) -> T_des_Drive decreases/1(Activate)
  v = const & phi_Acc = const/1(Activate) -> T_des_Drive = const/1(Activate)
  v increases & phi_Acc = const & T_des_Drive >= 0/1(Activate) -> T_des_Drive does not increase/1(Activate)
  Bus Creator/1 -> Test Info/1
  T_des_Drive does not increase/1(VF info) -> Bus Creator/4
  T_des_Drive = const/1(VF info) -> Bus Creator/3
  T_des_Drive decreases/1(VF info) -> Bus Creator/2
  T_des_Drive increases/1(VF info) -> Bus Creator/1
  v = const & phi_Acc increases & T_des_Drive < 0/1(Activate) -> "T_des_Drive decreases "/1(Activate)
  v = const & phi_Acc decreases & T_des_Drive < 0/1(Activate) -> "T_des_Drive increases "/1(Activate)
  "T_des_Drive decreases "/1(VF info) -> Bus Creator/5
  "T_des_Drive increases "/1(VF info) -> Bus Creator/6

== system LCTC_vTD8_Test_TC0_ref6_2007a/TestData/SR-PI-01.1 Brake Pedal recognition/Initialisation & Stabilisation ==
  Constant 1 : Constant  Value=0  OutDataType=sfix(16)  OutScaling=2^0
  Constant 2 : Constant  Value=0  OutDataType=sfix(16)  OutScaling=2^0
  Constant 3 : Constant  Value=0  OutDataType=sfix(16)  OutScaling=2^0
  v_Fzg neutral : Outport  OutDataType=sfix(16)  OutScaling=2^0
  phi_Acc neutral : Outport  Port=2  OutDataType=sfix(16)  OutScaling=2^0
  phi_Brake neutral : Outport  Port=3  OutDataType=sfix(16)  OutScaling=2^0
  wires:
  Constant 1/1 -> v_Fzg neutral/1  "Constant 1"
  Constant 2/1 -> phi_Acc neutral/1  "Constant 2"
  Constant 3/1 -> phi_Brake neutral/1  "Constant 3"

== system LCTC_vTD8_Test_TC0_ref6_2007a/TestData/SR-PI-01.1 Brake Pedal recognition/phi_Brake < ped_min ==
  Generate decrease 2 : Subsystem
  phi_Brake : Outport  OutDataType=sfix(16)  OutScaling=2^0
  wires:
  Generate decrease 2/1(phi_Brake) -> phi_Brake/1

== system LCTC_vTD8_Test_TC0_ref6_2007a/TestData/SR-PI-01.1 Brake Pedal recognition/phi_Brake >= ped_min ==
  Generate increase 2 : Subsystem
  phi_Brake : Outport  OutDataType=sfix(16)  OutScaling=2^0
  wires:
  Generate increase 2/1(phi_Brake) -> phi_Brake/1

== system LCTC_vTD8_Test_TC0_ref6_2007a/TestData/SR-PI-01.3 Acceleration Pedal recognition/Initialisation & Stabilisation ==
  Constant 1 : Constant  Value=0  OutDataType=sfix(16)  OutScaling=2^0
  Constant 2 : Constant  Value=0  OutDataType=sfix(16)  OutScaling=2^0
  Constant 3 : Constant  Value=0  OutDataType=sfix(16)  OutScaling=2^0
  v_Fzg neutral : Outport  OutDataType=sfix(16)  OutScaling=2^0
  phi_Acc neutral : Outport  Port=2  OutDataType=sfix(16)  OutScaling=2^0
  phi_Brake neutral : Outport  Port=3  OutDataType=sfix(16)  OutScaling=2^0
  wires:
  Constant 1/1 -> v_Fzg neutral/1  "Constant 1"
  Constant 2/1 -> phi_Acc neutral/1  "Constant 2"
  Constant 3/1 -> phi_Brake neutral/1  "Constant 3"

== system LCTC_vTD8_Test_TC0_ref6_2007a/TestData/SR-PI-01.3 Acceleration Pedal recognition/phi_Acc < ped_min ==
  Generate decrease 2 : Subsystem
  phi_Acc : Outport  OutDataType=sfix(16)  OutScaling=2^0
  wires:
  Generate decrease 2/1(phi_Acc) -> phi_Acc/1

== system LCTC_vTD8_Test_TC0_ref6_2007a/TestData/SR-PI-01.3 Acceleration Pedal recognition/phi_Acc >= ped_min ==
  Generate increase 2 : Subsystem
  phi_Acc : Outport  OutDataType=sfix(16)  OutScaling=2^0
  wires:
  Generate increase 2/1(phi_Acc) -> phi_Acc/1

== system LCTC_vTD8_Test_TC0_ref6_2007a/TestData/SR-PI-02.1 Brake pedal interpretation/Initialisation & Stabilisation ==
  Constant 1 : Constant  Value=0  OutDataType=sfix(16)  OutScaling=2^0
  Constant 2 : Constant  Value=0  OutDataType=sfix(16)  OutScaling=2^0
  Constant 3 : Constant  Value=0  OutDataType=sfix(16)  OutScaling=2^0
  v_Fzg neutral : Outport  OutDataType=sfix(16)  OutScaling=2^0
  phi_Acc neutral : Outport  Port=2  OutDataType=sfix(16)  OutScaling=2^0
  phi_Brake neutral : Outport  Port=3  OutDataType=sfix(16)  OutScaling=2^0
  wires:
  Constant 1/1 -> v_Fzg neutral/1  "Constant 1"
  Constant 2/1 -> phi_Acc neutral/1  "Constant 2"
  Constant 3/1 -> phi_Brake neutral/1  "Constant 3"

== system LCTC_vTD8_Test_TC0_ref6_2007a/TestData/SR-PI-02.1 Brake pedal interpretation/true ==
  phi_Acc random : Constant  Value=2  OutDataType=sfix(16)  OutScaling=2^0
  phi_Brake random : Constant  Value=0  OutDataType=sfix(16)  OutScaling=2^0
  v_Fzg random : Constant  OutDataType=sfix(16)  OutScaling=2^0
  v_Fzg : Outport  OutDataType=sfix(16)  OutScaling=2^0
  phi_Acc : Outport  Port=2  OutDataType=sfix(16)  OutScaling=2^0
  phi_Brake : Outport  Port=3  OutDataType=sfix(16)  OutScaling=2^0
  wires:
  v_Fzg random/1 -> v_Fzg/1  "v_Fzg"
  phi_Acc random/1 -> phi_Acc/1  "phi_Acc"
  phi_Brake random/1 -> phi_Brake/1  "phi_Brake"
